simulink model "test11_sub_named_System_diff"  (R2016b)
settings: Solver=VariableStepAuto  StartTime=0.0  StopTime=10.0  RelTol=1e-3
settings Model: Creator=gm  LastModifiedBy=gm

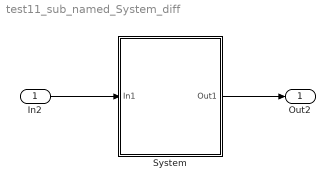
== system test11_sub_named_System_diff ==
  In2 : Inport
  System : Subsystem
  Out2 : Outport
  wires:
  In2/1 -> System/1(In1)
  System/1(Out1) -> Out2/1

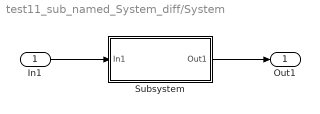
== system test11_sub_named_System_diff/System ==
  In1 : Inport
  Subsystem : Subsystem
  Out1 : Outport
  wires:
  In1/1 -> Subsystem/1(In1)
  Subsystem/1(Out1) -> Out1/1

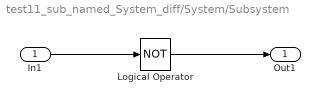
== system test11_sub_named_System_diff/System/Subsystem ==
  In1 : Inport
  Logical Operator : Logic  Operator=NOT  AllPortsSameDT=off  OutDataTypeStr=boolean
  Out1 : Outport
  wires:
  In1/1 -> Logical Operator/1
  Logical Operator/1 -> Out1/1
